simulink model "lab2"  (R2018b)
settings: Solver=VariableStepAuto  StartTime=0.0  StopTime=200  RelTol=1e-3
InitFcn:
  | %[num,den] = tfdata(C);
  | %num=cell2mat(num);
  | %kd=num(1,1);
  | %kp=num(1,2);
  | %ki=num(1,3);
  | s=.0177; % area
  | h=.108; % height
  | v0=h*s;%area*height
  | k=140*2*(sqrt(s*v0))
settings Model: Creator=exx241  LastModifiedBy=Matteo Cecamore

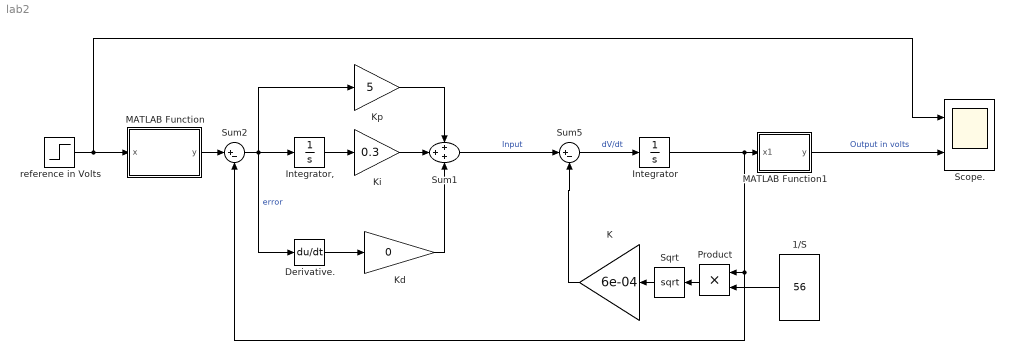
== system lab2 ==
  1/S : Constant  Value=56
  Derivative. : Derivative
  Integrator : Integrator  InitialCondition=.0013
  Integrator, : Integrator  UpperSaturationLimit=100  LowerSaturationLimit=-100
  K : Gain  Gain=6e-04
  Kd : Gain  Gain=0
  Ki : Gain  Gain=0.3
  Kp : Gain  Gain=5
  MATLAB Function : MATLAB Function  TreatAsAtomicUnit=on
  MATLAB Function1 : MATLAB Function  TreatAsAtomicUnit=on
  Product : Product
  Scope. : Scope  NumInputPorts=2
  Sqrt : Sqrt  SaturateOnIntegerOverflow=on
  Sum1 : Sum  Inputs=+++
  Sum2 : Sum  Inputs=|+-
  Sum5 : Sum  Inputs=|+-
  reference in Volts : Step  Time=.01  Before=6  After=6.5  SampleTime=0
  wires:
  Sum5/1 -> Integrator/1  "dV/dt"
  1/S/1 -> Product/2
  Product/1 -> Sqrt/1
  Sqrt/1 -> K/1
  K/1 -> Sum5/2
  Kp/1 -> Sum1/1
  Ki/1 -> Sum1/2
  Kd/1 -> Sum1/3
  Sum2/1 -> Derivative./1, Integrator,/1, Kp/1  "error"
  Derivative./1 -> Kd/1
  Integrator,/1 -> Ki/1
  reference in Volts/1 -> MATLAB Function/1(x), Scope./1
  MATLAB Function/1(y) -> Sum2/1
  MATLAB Function1/1(y) -> Scope./2  "Output in volts"
  Integrator/1 -> MATLAB Function1/1(x1), Sum2/2, Product/1
  Sum1/1 -> Sum5/1  "Input"

== matlab function lab2/MATLAB Function1 ==
  data: x1 input; y output
function y = fcn(x1)
x=x1/.0177;  %volume to height or level conversion
p1 =     1.9e+06; p2 =  -1.193e+06;p3 =   2.812e+05;p4 =  -3.063e+04  
p5 =        1248;p6 =       76.14;p7 =     0.01028; 
y = p1*x^6 + p2*x^5 + p3*x^4 + p4*x^3 + p5*x^2 + p6*x + p7;

== matlab function lab2/MATLAB Function ==
  data: x input; y output
function y = fcn(x)
p1=4.455e-06;p2 =  -0.0001234;p3 =    0.001272;p4 =   -0.005882;  
p5 =     0.01189;  p6 =    0.002743;p7 =   0.0003275; 
y1 = p1*x^6 + p2*x^5 + p3*x^4 + p4*x^3 + p5*x^2 + p6*x + p7;
y=y1*.0177;
